simulink model "shell_elec_electric_vehicle"  (R2016b)
settings: Solver=FixedStepAuto  StartTime=0.0  StopTime=200  RelTol=1e-3  AbsTol=1e-3
PreLoadFcn:
  | % Simulation parameters
  | dt = 0.01;
  | 
  | % Battery cell parameters
  | ssc_lithium_cell_1RC_ini
  | 
  | % Motor parameters
  | max_torque = 220;
  | max_power = 50e3;
  | 
  | % Vehicle parameters
  | vehicle_mass = 1000;
  | wheel_radius = 0.25;
  | area = 5;
  | drag_coefficient = 0.25;
  | air_density = 1.225;
  | gravity = 9.81;
  | rolling_res_ratio = 0.015;
  | 
  | % Differential drive parameters
  | gear_ratio = 6;
  | 
  | % Simplified braking system parameters
  | force_max_pedal = 500;
  | braking_torque_to_pedal_force_ratio = -4;
  | 
  | % Vehicle controller parameters
  | hill_hold_max_speed = 0.5;
  | 
  | % Water properties for cooling circuit
  | load WaterProperties
values from neighbouring files (symbols this model uses):
  C1_LUT = [1913.6 12447 30609 ... (first row only)    [shell_elec_electric_vehicle_settings.m]
  Capacity_LUT = [28.0081 27.625 27.6392]    [shell_elec_electric_vehicle_settings.m]
  cell_mass = 1    [shell_elec_electric_vehicle_settings.m]
  Qe_init = 15.6845    [shell_elec_electric_vehicle_settings.m]
  R0_LUT = [0.0117 0.0085 0.009 ... (first row only)    [shell_elec_electric_vehicle_settings.m]
  R1_LUT = [0.0109 0.0029 0.0013 ... (first row only)    [shell_elec_electric_vehicle_settings.m]
  T_init = 293.15    [shell_elec_electric_vehicle_settings.m]
undefined symbols (not defined in the file or in its folder): DiscIntNeverNeededParam, sigbuilder_block
undefined symbols (not defined in the file): cell_Cp_heat, Em_LUT, SOC_LUT, Temperature_LUT
libraries: fl_lib x82, nesl_utility x12, LiBatteryElements_lib x4, elec_lib x2, instrumentlib x2, simulink_extras x1, simulink x1
Description:
  | Electric Vehicle Configured for HIL
  | 
  | This example shows an electric vehicle model suitable for
  | Hardware-In-the-Loop (HIL) deployment. Energy-based modeling
  | is used to avoid high-frequency switching, and solvers set for
  | fixed-step simulation.
  | 
  | The test run shows the vehicle accelerating to a steady speed up
  | an incline followed by a period of descent during which electrical
  | power is returned to the battery.
  | 
  | Copyright 2008-2016 The MathWorks, Inc.
settings Model: Creator=MathWorks  LastModifiedBy=eliya
settings SolverCC: InitialStep=1e-3
settings DataIOCC: LimitDataPoints=on  SaveFormat=Array  InspectSignalLogs=on
settings OptimizationCC: BlockReduction=off  BooleanDataType=off  LifeSpan=inf
settings DebuggingCC: SaveWithParameterizedLinksMsg=none  UnderspecifiedInitializationDetection=Classic  MergeDetectMultiDrivingBlocksExec=none  SignalResolutionControl=TryResolveAllWithWarning  AllowSymbolicDim=off  SFUnexpectedBacktrackingDiag=warning  SFNoUnconditionalDefaultTransitionDiag=warning  SFExecutionAtInitializationDiag=none
settings HardwareCC: ProdBitPerPointer=32  ProdBitPerSizeT=32  ProdBitPerPtrDiffT=32  ProdLargestAtomicFloat=None  ProdIntDivRoundTo=Undefined  ProdEndianess=Unspecified  ProdWordSize=32  ProdHWDeviceType=32-bit Generic  TargetUnknown=on
settings ModelReferenceCC: PropagateSignalLabelsOutOfModel=off
settings GRTTargetCC: TargetLangStandard=C89/C90 (ANSI)  GeneratePreprocessorConditionals=Disable all
settings ConfigComp: CovMetricSettings=dw  CovHtmlReporting=on  CovSaveCumulativeToWorkspaceVar=on  CovSaveSingleToWorkspaceVar=on  CovExternalEMLEnable=off  CovSFcnEnable=off
settings SimscapeCC: SimscapeLogType=all  SimscapeLogName=simlog_elec_electric_vehicle  SimscapeLogDataHistory=10000

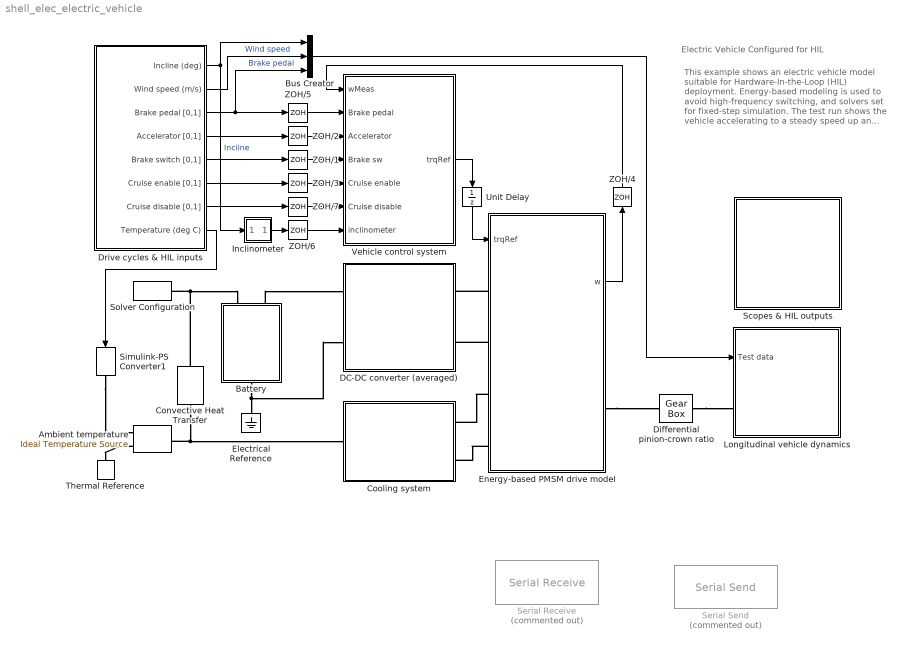
== system shell_elec_electric_vehicle ==
  note: Electric Vehicle Configured for HIL
  note: This example shows an electric vehicle model suitable for Hardware-In-the-Loop (HIL) deployment. Energy-based modeling is used to avoid high-frequency switching, and solvers set for fixed-step simulation.
      |
      | The test run shows the vehicle accelerating to a steady speed up an incline followed by a period of descent during which electrical power is returned to the battery.
  Ambient temperature : fl_lib/Thermal/Thermal Sources/Ideal Temperature Source
  Battery : Subsystem  mask(Lithium cell (one RC-branch equivalent circuit)){Nseries=50, Nparallel=10, Qe_init=Qe_init, T_init=T_init, Capacity_LUT=Capacity_LUT, Em_LUT=Em_LUT, R0_LUT=R0_LUT, R1_LUT=R1_LUT, C1_LUT=C1_LUT, cell_mass=cell_mass, cell_Cp_heat=cell_Cp_heat, SOC_LUT=SOC_LUT, Temperature_LUT=Temperature_LUT}
      mask prompts: Nseries "Number of series-connected cells"; Nparallel "Number of parallel sets of series-connected cells"; Qe_init "Initial cell charge deficit (A*hr)"; T_init "Initial cell temperature (K)"; Capacity_LUT "Capacity (A*hr, 1xN table)"; Em_LUT "Em open-circuit voltage, Em (volts, MxN table)"; R0_LUT "R0 terminal resistance (ohms, MxN table)"; R1_LUT "R1 cell resistance (ohms, MxN table)"; C1_LUT "C1 capacitance (farads, MxN table)"; cell_mass "Cell mass (kg)"; cell_Cp_heat "Cell specific heat (J/kg/K)"; SOC_LUT "SOC table breakpoints (Mx1 array)"; Temperature_LUT "Temperature table breakpoints (K, 1xN array)"
      mask Display:
      | % Battery icon
      | plot([2.5 1.3],[0 0])
      | plot([-0.6 -1.6 -1.6 -2.5],[0 0 -0.8 -0.8])
      | patch([1 1 -1 -1]*0.15+1.3,[-1 1 1 -1]*0.4,[0;0;0]);
      | patch([1 1 -1 -1]*0.15+0.0,[-1 1 1 -1]*0.4,[0;0;0]);
      | patch([1 1 -1 -1]*0.15+0.7,[-1 1 1 -1]*0.8,[0;0;0]);
      | patch([1 1 -1 -1]*0.15-0.6,[-1 1 1 -1]*0.8,[0;0;0]);
      | % Thermal port
      | plot([-1.6,-1.3],[1.2,1.2])
      | plot([-1.6,-1.3],[0.5,0.5])
      | plot([-1.6,-2.5],[0.8,0.8])
      | plot(0.2*sin(0:2*pi/50:2*pi)-1.6,0.35*cos(0:2*pi/50:2*pi)+0.85)
      | plot(0.2*sin(0:2*pi/50:pi)-1.3,0.35*cos(0:2*pi/50:pi)+0.85)
      | 
      | % Plot points to set plot range
      | color('white');plot(2.5,1.5);plot(-2.5,-1.5)
      | 
      | color('red')
      | port_label('LConn',1,'H')
      | port_label('LConn',2,'+')
      | port_label('RConn',1,'-')
  Bus Creator : BusCreator  Inputs=3
  Convective Heat Transfer : fl_lib/Thermal/Thermal Elements/Convective Heat Transfer  area=cell_area m^2  heat_tr_coeff=h_conv W/(m^2 * K)  Q_specify=off  Q_priority=High  Q=0 J/s  T_specify=off  T_priority=High  T=0 K
  Cooling system : Subsystem
  DC-DC converter (averaged) : Subsystem
  Differential pinion-crown ratio : fl_lib/Mechanical/Mechanisms/Gear Box  ratio=gear_ratio  t_in_specify=off  t_in_priority=High  t_in=0 N*m  t_out_specify=off  t_out_priority=High  t_out=0 N*m
  Drive cycles & HIL inputs : Subsystem  Tag=STV Subsys  LoadFcn=sigbuilder_block('load',[6 33 1428 678 ]);  StartFcn=sigbuilder_block('start');  StopFcn=sigbuilder_block('stop');  ClipboardFcn=sigbuilder_block('clipboard');  mask(Sigbuilder block){tuvar=[0:10]}
      mask help: Simulink:masks:SigbuilderBlock_MD
      mask init:
      | if ~strcmp(get_param(bdroot(gcbh),'SimulationStatus'),'stopped') tuvar = sigbuilder_block('maskInit'); end
      settings: CopyFcn=sigbuilder_block('copy');  DeleteFcn=sigbuilder_block('delete');  ModelCloseFcn=sigbuilder_block('modelClose');  PreSaveFcn=sigbuilder_block('preSave');  PauseFcn=sigbuilder_block('pause');  ContinueFcn=sigbuilder_block('continue');  NameChangeFcn=sigbuilder_block('namechange');  OpenFcn=sigbuilder_block('open',[6 33 1428 678 ]);  CloseFcn=sigbuilder_block('close');
      mask Display: plot(0, 0, 100, 100,[2, 2, 32, 32, 2], [68, 8, 8, 68, 68],[32, 2], [38, 38], [32, 19, 2],[53, 60, 44], [32, 17, 17, 2],[16, 16, 31, 31]);txt = getActiveGroup(gcbh);text(2, 100, txt,'verticalAlignment', 'top');
  Electrical Reference : fl_lib/Electrical/Electrical Elements/Electrical Reference
  Energy-based PMSM drive model : Subsystem  VariantControl=Variant1
  Inclinometer : Subsystem
  Longitudinal vehicle dynamics : Subsystem
  Scopes & HIL outputs : Subsystem
  Serial Receive : instrumentlib/Serial Receive  Commented=on  ComPortMenu=<Please select a port...>  ComPort=<Please select a port...>  Terminator=<none>  DataSize=[1 1]  DataType=uint8  EnableBlockingMode=on  ActionDataUnavailable=Output last received value  CustomValue=0  SampleTime=0.01
  Serial Send : instrumentlib/Serial Send  Commented=on  ComPortMenu=<Please select a port...>  ComPort=<Please select a port...>  Terminator=<none>  EnableBlockingMode=on
  Simulink-PS Converter1 : nesl_utility/Simulink-PS Converter  PhysicalDomain=network_engine_domain  SubClassName=ps_input  LeftPortType=input  RightPortType=output  PseudoPeriodic=off  Frequencies=[]  NoiseDistribution=none  NoiseParameters=[]  Unit=degC  AffineConversion=on  InputFiltering=off  SimscapeFilterOrder=1  InputFilterTimeConstant=.001  UdotUserProvided=1
  Solver Configuration : nesl_utility/Solver Configuration  PhysicalDomain=network_engine_domain  SubClassName=solver  LeftPortType=input  RightPortType=generic  Accelerate=off  Tones=[]  Harmonics=[]  SimulateNoise=off  Profile=off  UseLocalSampling=off  EnableSwitchedLinearOptims=on  FrequencyDomain=off  UseCCode=off  RelTol=0.001  AbsTol=1e-06  MinStep=1e-09  ToWorkspace=off  RevertToSquareIcSolve=off  NumHomotopyIterations=100  PhasorMode=off  PhasorModeNumHarmonics=1  OverrideAbsTol=off  DoDC=off  ResidualTolerance=1e-9  UseLocalSolver=on  LocalSolverChoice=NE_BACKWARD_EULER_ADVANCER  LocalSolverSampleTime=dt  DoFixedCost=on  MaxNonlinIter=3  MaxModeIter=2  LinearAlgebra=Sparse  DelaysMemoryBudget=1024  AutomaticFiltering=on  FilteringTimeConstant=0.001
  Thermal Reference : fl_lib/Thermal/Thermal Elements/Thermal Reference
  Unit Delay : UnitDelay  SampleTime=dt
  Vehicle control system : Subsystem
  ZOH/{1..7} (7 alike) : ZeroOrderHold  SampleTime=dt
  wires:
  Drive cycles & HIL inputs/8(Temperature (deg C)) -> Simulink-PS Converter1/1
  Drive cycles & HIL inputs/1(Incline (deg)) -> Bus Creator/1, Inclinometer/1(a)  "Incline"
  Drive cycles & HIL inputs/2(Wind speed (m/s)) -> Bus Creator/2  "Wind speed"
  ZOH/2/1 -> Vehicle control system/3(Accelerator)
  Drive cycles & HIL inputs/4(Accelerator [0,1]) -> ZOH/2/1
  ZOH/3/1 -> Vehicle control system/5(Cruise enable)
  Drive cycles & HIL inputs/6(Cruise enable [0,1]) -> ZOH/3/1
  ZOH/5/1 -> Vehicle control system/2(Brake pedal)
  ZOH/1/1 -> Vehicle control system/4(Brake sw)
  ZOH/6/1 -> Vehicle control system/7(inclinometer)
  ZOH/7/1 -> Vehicle control system/6(Cruise disable)
  Drive cycles & HIL inputs/3(Brake pedal [0,1]) -> ZOH/5/1, Bus Creator/3  "Brake pedal"
  ZOH/4/1 -> Vehicle control system/1(wMeas)
  Drive cycles & HIL inputs/5(Brake switch [0,1]) -> ZOH/1/1
  Drive cycles & HIL inputs/7(Cruise disable [0,1]) -> ZOH/7/1
  Inclinometer/1(y) -> ZOH/6/1
  Vehicle control system/1(trqRef) -> Unit Delay/1
  Unit Delay/1 -> Energy-based PMSM drive model/1(trqRef)
  Energy-based PMSM drive model/1(w) -> ZOH/4/1
  Bus Creator/1 -> Longitudinal vehicle dynamics/1(Test data)
  connections:
  Ambient temperature/RConn2 -- Thermal Reference/LConn1
  Simulink-PS Converter1/RConn1 -- Ambient temperature/RConn1
  Convective Heat Transfer/RConn1 -- Solver Configuration/RConn1 -- Battery/LConn1
  Battery/RConn1 -- DC-DC converter (averaged)/LConn2 -- Electrical Reference/LConn1
  Battery/LConn2 -- DC-DC converter (averaged)/LConn1
  Differential pinion-crown ratio/RConn1 -- Longitudinal vehicle dynamics/LConn1
  Energy-based PMSM drive model/LConn1 -- DC-DC converter (averaged)/RConn1
  Energy-based PMSM drive model/LConn2 -- DC-DC converter (averaged)/RConn2
  Energy-based PMSM drive model/RConn1 -- Differential pinion-crown ratio/LConn1
  Convective Heat Transfer/LConn1 -- Ambient temperature/LConn1 -- Cooling system/LConn1
  Energy-based PMSM drive model/LConn4 -- Cooling system/RConn2
  Energy-based PMSM drive model/LConn3 -- Cooling system/RConn1

== system shell_elec_electric_vehicle/Battery ==
  note: Scale up voltage drop to total of Ns series-connected cells
  Controlled Voltage Source : fl_lib/Electrical/Electrical Sources/Controlled Voltage Source
  Electrical model for Np parallel-connected cells : Subsystem
  Ns : fl_lib/Physical Signals/Functions/PS Gain  gain=Nseries
  Ns-1 : fl_lib/Physical Signals/Functions/PS Gain  gain=(Nseries-1)
  Thermal Model : Subsystem
  Voltage Sensor : fl_lib/Electrical/Electrical Sensors/Voltage Sensor
  - : PMIOPort  Tag=PMCPort  Port=1  Side=Right
  H : PMIOPort  Tag=PMCPort  Port=2  Side=Left
  + : PMIOPort  Tag=PMCPort  Port=3  Side=Left
  connections:
  Controlled Voltage Source/RConn2 -- -/RConn1
  Ns-1/RConn1 -- Controlled Voltage Source/RConn1
  +/RConn1 -- Electrical model for Np parallel-connected cells/RConn1 -- Voltage Sensor/LConn1
  Voltage Sensor/RConn1 -- Ns-1/LConn1
  Controlled Voltage Source/LConn1 -- Electrical model for Np parallel-connected cells/RConn2 -- Voltage Sensor/RConn2
  H/RConn1 -- Thermal Model/LConn2
  Thermal Model/RConn1 -- Electrical model for Np parallel-connected cells/LConn2
  Electrical model for Np parallel-connected cells/LConn1 -- Ns/LConn1
  Ns/RConn1 -- Thermal Model/LConn1

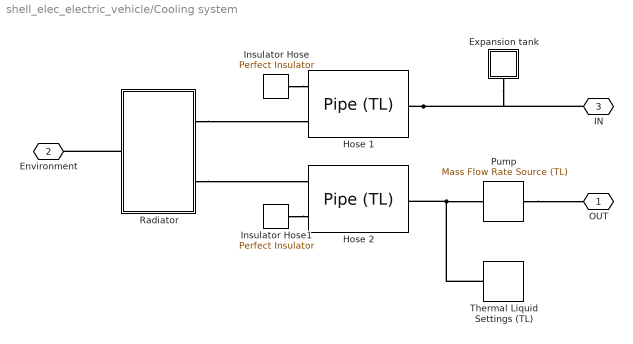
== system shell_elec_electric_vehicle/Cooling system ==
  Expansion tank : Subsystem
  Hose 1 : fl_lib/Thermal Liquid/Elements/Pipe (TL)  dynamic_compressibility=1  inertia=0  length=500 mm  area=pi*25^2 mm^2  Dh=50 mm  length_add=500 mm  roughness=1.5e-5 m  Re_lam=2e+3  Re_tur=4e+3  shape_factor=64  Nu_lam=3.66  p0=1 atm  T0=20 degC  mdot0=0.1 kg/s
  Hose 2 : fl_lib/Thermal Liquid/Elements/Pipe (TL)  dynamic_compressibility=1  inertia=0  length=500 mm  area=pi*25^2 mm^2  Dh=50 mm  length_add=500 mm  roughness=1.5e-5 m  Re_lam=2e+3  Re_tur=4e+3  shape_factor=64  Nu_lam=3.66  p0=1 atm  T0=20 degC  mdot0=0.1 kg/s
  Insulator Hose : fl_lib/Thermal/Thermal Elements/Perfect Insulator  T_specify=off  T_priority=High  T=0 K
  Insulator Hose1 : fl_lib/Thermal/Thermal Elements/Perfect Insulator  T_specify=off  T_priority=High  T=0 K
  Pump : fl_lib/Thermal Liquid/Sources/Mass Flow Rate Source (TL)  commanded_mass_flow=0.2 kg/s  area=pi*25^2 mm^2  length=1e-1 m
  Radiator : Subsystem
  Thermal Liquid Settings (TL) : fl_lib/Thermal Liquid/Utilities/Thermal Liquid Settings (TL)  pT_region_flag=0  T_min=273.16 K  T_max=373.16 K  p_min=0.1 bar  p_max=500 bar  T_TLU=T K  p_TLU=p Pa  pT_validity_TLU=ones(11, 12)  rho_TLU=rho kg/m^3  u_TLU=u J/g  nu_TLU=nu cm^2/s  cp_TLU=Cp J/K/g  k_TLU=k mW/m/K  beta_TLU=beta Pa  alpha_TLU=alpha 1/K  p_atm=1 atm
  OUT : PMIOPort  Port=1  Side=Right
  Environment : PMIOPort  Port=2  Side=Left
  IN : PMIOPort  Port=3  Side=Right
  connections:
  Insulator Hose1/LConn1 -- Hose 2/LConn2
  Insulator Hose/LConn1 -- Hose 1/LConn2
  Radiator/LConn1 -- Environment/RConn1
  Thermal Liquid Settings (TL)/RConn1 -- Pump/LConn1 -- Hose 2/RConn1
  Radiator/RConn1 -- Hose 1/LConn1
  Radiator/RConn2 -- Hose 2/LConn1
  Pump/RConn1 -- OUT/RConn1
  Hose 1/RConn1 -- Expansion tank/RConn1 -- IN/RConn1

== system shell_elec_electric_vehicle/DC-DC converter (averaged) ==
  Battery sensors : Subsystem
  DC-DC Converter : elec_lib/Sources/DC-DC Converter  v_ref=400 V  P_rated=60 kW  droop_param=2  droop=0.1 V/A  droop_percent=1  reversible=1  efficiency=98  P_fixed=100 W  model_dynamics=0  tau=0.02 s  v_ini=400 V  i1_max=1000 A  fault_condition=1  fault_threshold=0.5  R_fixed=100 Ohm  R_out=0.1 Ohm  fault_sign=1
  No faults : fl_lib/Physical Signals/Sources/PS Constant  constant=0
  Resistor : fl_lib/Electrical/Electrical Elements/Resistor  R=0.002 Ohm  i_specify=off  i_priority=None  i=0 A  v_specify=off  v_priority=None  v=0 V
  Vbat+ : PMIOPort  Port=1  Side=Left
  V+ : PMIOPort  Tag=PMCPort  Port=2  Side=Right
  Vbat- : PMIOPort  Port=3  Side=Left
  V- : PMIOPort  Tag=PMCPort  Port=4  Side=Right
  connections:
  No faults/RConn1 -- DC-DC Converter/LConn3
  DC-DC Converter/RConn2 -- V-/RConn1 -- DC-DC Converter/LConn2 -- Battery sensors/LConn1 -- Vbat-/RConn1
  Vbat+/RConn1 -- Battery sensors/RConn1
  Battery sensors/RConn2 -- DC-DC Converter/LConn1
  DC-DC Converter/RConn1 -- Resistor/LConn1
  Resistor/RConn1 -- V+/RConn1

== system shell_elec_electric_vehicle/Drive cycles & HIL inputs ==
  Demux : Demux  Tag=STV Demux  Outputs=8
  FromWs : FromWorkspace  Tag=STV FromWs  VariableName=tuvar  SampleTime=0.01
      SigBuilderData=|
      | common.afterFinalStr = 'Extrapolate'
      | common.sampleTime = '0.01'
      | dataSet.timeRange = [0 200]
      | dataSet.name = 'Test 1'
      | sbobj.Name = 'Signal Builder'
      | sbobj.Groups.Name = 'Test 1'
      | sbobj.Groups.Signals(1).Name = 'Incline (deg)'
      | sbobj.Groups.Signals(1).XData = [0 100 200]
      | sbobj.Groups.Signals(1).YData = [0 0 0]
      | sbobj.Groups.Signals(2).Name = 'Wind speed (m/s)'
      | sbobj.Groups.Signals(2).XData = [0 200]
      | sbobj.Groups.Signals(2).YData = [0 0]
      | sbobj.Groups.Signals(3).Name = 'Brake pedal [0,1]'
      | sbobj.Groups.Signals(3).XData = [0 180 180 200]
      | sbobj.Groups.Signals(3).YData = [0 0 1 1]
      | sbobj.Groups.Signals(4).Name = 'Accelerator [0,1]'
      | sbobj.Groups.Signals(4).XData = [0 0.1 0.3 7.5 50 200]
      | sbobj.Groups.Signals(4).YData = [0 0 0 1 0 0]
      | sbobj.Groups.Signals(5).Name = 'Brake switch [0,1]'
      | sbobj.Groups.Signals(5).XData = [0 180 180 200]
      | sbobj.Groups.Signals(5).YData = [0 0 1 1]
      | sbobj.Groups.Signals(6).Name = 'Cruise enable [0,1]'
      | sbobj.Groups.Signals(6).XData = [0 8 8 10 10 200]
      | sbobj.Groups.Signals(6).YData = [0 0 1 1 0 0]
      | sbobj.Groups.Signals(7).Name = 'Cruise disable [0,1]'
      | sbobj.Groups.Signals(7).XData = [0 200]
      | sbobj.Groups.Signals(7).YData = [0 0]
      | sbobj.Groups.Signals(8).Name = 'Temperature (deg C)'
      | sbobj.Groups.Signals(8).XData = [0 200]
      | sbobj.Groups.Signals(8).YData = [25 25]
      | sbobj.Groups.TimeRange = [0 200]
  Incline (deg) : Outport  Tag=STV Outport
  Wind speed (m/s) : Outport  Tag=STV Outport  Port=2
  Brake pedal [0,1] : Outport  Tag=STV Outport  Port=3
  Accelerator [0,1] : Outport  Tag=STV Outport  Port=4
  Brake switch [0,1] : Outport  Tag=STV Outport  Port=5
  Cruise enable [0,1] : Outport  Tag=STV Outport  Port=6
  Cruise disable [0,1] : Outport  Tag=STV Outport  Port=7
  Temperature (deg C) : Outport  Tag=STV Outport  Port=8
  wires:
  FromWs/1 -> Demux/1
  Demux/1 -> Incline (deg)/1
  Demux/2 -> Wind speed (m/s)/1
  Demux/3 -> Brake pedal [0,1]/1
  Demux/4 -> Accelerator [0,1]/1
  Demux/5 -> Brake switch [0,1]/1
  Demux/6 -> Cruise enable [0,1]/1
  Demux/7 -> Cruise disable [0,1]/1
  Demux/8 -> Temperature (deg C)/1

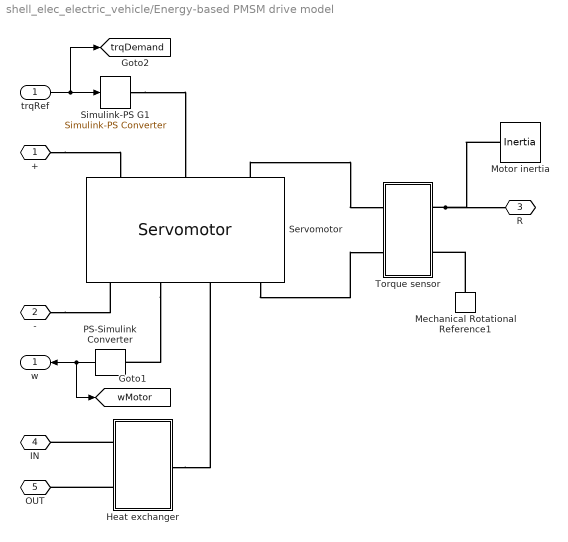
== system shell_elec_electric_vehicle/Energy-based PMSM drive model ==
  trqRef : Inport
  Heat exchanger : Subsystem
  Mechanical Rotational Reference1 : fl_lib/Mechanical/Rotational Elements/Mechanical Rotational Reference
  Motor inertia : fl_lib/Mechanical/Rotational Elements/Inertia  inertia=0.02 kg*m^2  w_specify=on  w_priority=High  w=0 rpm  t_specify=off  t_priority=High  t=0 N*m
  PS-Simulink Converter : nesl_utility/PS-Simulink Converter  PhysicalDomain=network_engine_domain  SubClassName=ps_output  LeftPortType=input  RightPortType=output  PseudoPeriodic=off  Frequencies=[]  Unit=rad/s  AffineConversion=off
  Servomotor : elec_lib/Actuators & Drivers/Rotational Actuators/Servomotor  torque_speed_param=2  w_t=[ 0 3.75e+3 7.5e+3 8e+3 ] rpm  T_t=[max_torque max_torque max_torque 0] N*m  torque_max=max_torque N*m  power_max=max_power W  Tc=0.02 s  losses_param=1  eff=96  w_eff=1500 rpm  T_eff=50 N*m  Piron=200 W  Pbase=0 W  w_eff_vec=[-8000 -4000 0 4000 8000] rpm  T_eff_vec=[0 0.03 0.06 0.09] N*m  losses_mat=[1.49 1.67 2.21 3.10; 0.42 0.69 1.14 2.03; 0.06 0.24 0.78 1.68; 0.42 0.69 1.14 2.03; 1.49 1.67 2.21 3.10] W  efficiency_mat=[95 95 95 95; 95 95 95 95; 95 95 95 95; 95 95 95 95; 95 95 95 95]  Res=0 Ohm  J=0 kg*m^2  lam=1e-5 N*m/(rad/s)  speed0=0 rpm  alpha=0.00393 1/K  Tmeas=25 degC  Tmeas2=125 degC  losses_mat_T2=[1.49 1.74 2.49 3.74;0.42 0.67 1.42 2.67;0.06 0.31 1.06 2.31;0.42 0.67 1.42 2.67;1.49 1.74 2.49 3.74] W  efficiency_mat_T2=[95 95 95 95; 95 95 95 95; 95 95 95 95; 95 95 95 95; 95 95 95 95]  thermal_mass=1500 J/K  initial_temperature=20 degC  fault_condition=1  fault_threshold=0.5
  Simulink-PS G1 : nesl_utility/Simulink-PS Converter  PhysicalDomain=network_engine_domain  SubClassName=ps_input  LeftPortType=input  RightPortType=output  PseudoPeriodic=off  Frequencies=[]  NoiseDistribution=none  NoiseParameters=[]  Unit=1  AffineConversion=off  InputFiltering=off  SimscapeFilterOrder=1  InputFilterTimeConstant=1e-6  UdotUserProvided=1
  Torque sensor : Subsystem
  + : PMIOPort  Port=1  Side=Left
  - : PMIOPort  Port=2  Side=Left
  R : PMIOPort  Port=3  Side=Right
  IN : PMIOPort  Port=4  Side=Left
  OUT : PMIOPort  Port=5  Side=Left
  w : Outport
  tag scope: trqDemand=global, wMotor=global
  wires:
  PS-Simulink Converter/1 -> w/1, [wMotor]
  trqRef/1 -> Simulink-PS G1/1, [trqDemand]
  connections:
  Servomotor/RConn2 -- PS-Simulink Converter/LConn1
  Simulink-PS G1/RConn1 -- Servomotor/LConn2
  -/RConn1 -- Servomotor/RConn1
  +/RConn1 -- Servomotor/LConn1
  Heat exchanger/LConn1 -- IN/RConn1
  Heat exchanger/LConn2 -- OUT/RConn1
  Heat exchanger/RConn1 -- Servomotor/RConn3
  Servomotor/LConn3 -- Torque sensor/LConn1
  Servomotor/RConn4 -- Torque sensor/LConn2
  Mechanical Rotational Reference1/LConn1 -- Torque sensor/RConn2
  Torque sensor/RConn1 -- R/RConn1 -- Motor inertia/LConn1

== system shell_elec_electric_vehicle/Inclinometer ==
  a : Inport
  Trigonometric Function : Trigonometry
  d2r : Gain  Gain=pi/180
  g : Gain  Gain=gravity
  y : Outport
  wires:
  Trigonometric Function/1 -> g/1
  a/1 -> d2r/1
  d2r/1 -> Trigonometric Function/1
  g/1 -> y/1

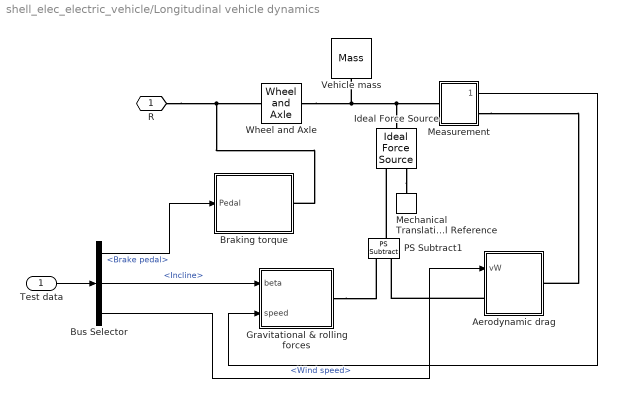
== system shell_elec_electric_vehicle/Longitudinal vehicle dynamics ==
  Test data : Inport
  Aerodynamic drag : Subsystem
  Braking torque : Subsystem
  Bus Selector : BusSelector  OutputSignals=Brake pedal,Incline,Wind speed
  Gravitational & rolling forces : Subsystem
  Ideal Force Source : fl_lib/Mechanical/Mechanical Sources/Ideal Force Source
  Measurement : Subsystem
  Mechanical Translational Reference : fl_lib/Mechanical/Translational Elements/Mechanical Translational Reference
  PS Subtract1 : fl_lib/Physical Signals/Functions/PS Subtract
  Vehicle mass : fl_lib/Mechanical/Translational Elements/Mass  mass=vehicle_mass kg  v_specify=off  v_priority=High  v=0 m/s  f_specify=off  f_priority=High  f=0 N
  Wheel and Axle : fl_lib/Mechanical/Mechanisms/Wheel and Axle  R=wheel_radius m  or=1  t_specify=off  t_priority=High  t=0 N*m  f_specify=off  f_priority=High  f=0 N
  R : PMIOPort  Port=1  Side=Left
  wires:
  Test data/1 -> Bus Selector/1
  Bus Selector/1 -> Braking torque/1(Pedal)  "<Brake pedal>"
  Bus Selector/2 -> Gravitational & rolling forces/1(beta)  "<Incline>"
  Bus Selector/3 -> Aerodynamic drag/1(vW)  "<Wind speed>"
  Measurement/1(speed) -> Gravitational & rolling forces/2(speed)
  connections:
  Ideal Force Source/RConn2 -- Mechanical Translational Reference/LConn1
  R/RConn1 -- Braking torque/RConn1 -- Wheel and Axle/LConn1
  PS Subtract1/RConn1 -- Ideal Force Source/RConn1
  Gravitational & rolling forces/RConn1 -- PS Subtract1/LConn1
  Aerodynamic drag/LConn1 -- PS Subtract1/LConn2
  Wheel and Axle/RConn1 -- Measurement/LConn1 -- Ideal Force Source/LConn1 -- Vehicle mass/LConn1
  Measurement/RConn1 -- Aerodynamic drag/RConn1

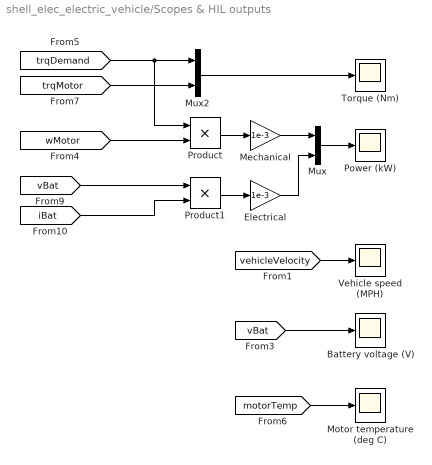
== system shell_elec_electric_vehicle/Scopes & HIL outputs ==
  " Electrical " : Gain  Gain=1e-3
  Battery voltage (V) : Scope
  Mechanical : Gain  Gain=1e-3
  Motor temperature (deg C) : Scope
  Mux : Mux  Inputs=2
  Mux2 : Mux  Inputs=2
  Power (kW) : Scope
  Product : Product
  Product1 : Product
  Torque (Nm) : Scope
  Vehicle speed (MPH) : Scope
  wires:
  [wMotor] -> Product/2
  [trqDemand] -> Product/1, Mux2/1
  [vehicleVelocity] -> Vehicle speed (MPH)/1
  [vBat] -> Battery voltage (V)/1
  Product/1 -> Mechanical/1
  [motorTemp] -> Motor temperature (deg C)/1
  [trqMotor] -> Mux2/2
  [vBat] -> Product1/1
  [iBat] -> Product1/2
  Product1/1 -> " Electrical "/1
  Mechanical/1 -> Mux/1
  " Electrical "/1 -> Mux/2
  Mux/1 -> Power (kW)/1
  Mux2/1 -> Torque (Nm)/1

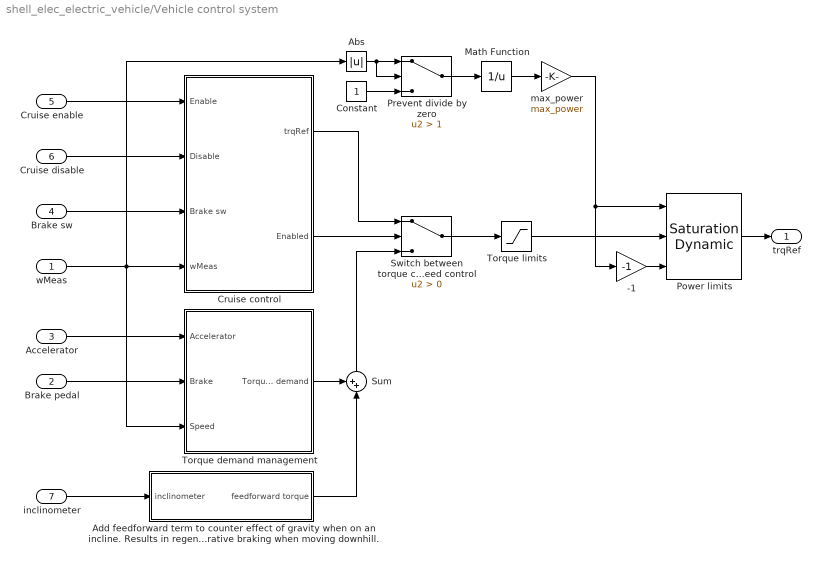
== system shell_elec_electric_vehicle/Vehicle control system ==
  wMeas : Inport
  Brake pedal : Inport  Port=2
  Accelerator : Inport  Port=3
  Brake sw : Inport  Port=4
  Cruise enable : Inport  Port=5
  Cruise disable : Inport  Port=6
  inclinometer : Inport  Port=7
  -1 : Gain  Gain=-1
  Abs : Abs
  Add feedforward term to counter effect of gravity when on an incline. Results in regenerative braking when moving downhill. : Subsystem
  Constant : Constant
  Cruise control : Subsystem
  Math Function : Math  Operator=reciprocal  SaturateOnIntegerOverflow=on
  Power limits : simulink/Discontinuities/Saturation Dynamic  OutMin=[]  OutMax=[]  OutDataTypeStr=Inherit: Same as second input  OutDataType=fixdt(1, 16)  OutScaling=2^-10  DoSatur=off
  Prevent divide by zero : Switch  Criteria=u2 > Threshold  Threshold=1
  Sum : Sum  Inputs=++|
  Switch between torque control and speed control : Switch  Criteria=u2 > Threshold
  Torque limits : Saturate  UpperLimit=max_torque  LowerLimit=-max_torque
  Torque demand management : Subsystem
  max_power : Gain  Gain=max_power
  trqRef : Outport
  wires:
  Switch between torque control and speed control/1 -> Torque limits/1
  Cruise enable/1 -> Cruise control/1(Enable)
  wMeas/1 -> Abs/1, Torque demand management/3(Speed), Cruise control/4(wMeas)
  Cruise control/1(trqRef) -> Switch between torque control and speed control/1
  Cruise control/2(Enabled) -> Switch between torque control and speed control/2
  Cruise disable/1 -> Cruise control/2(Disable)
  Brake sw/1 -> Cruise control/3(Brake sw)
  Accelerator/1 -> Torque demand management/1(Accelerator)
  Brake pedal/1 -> Torque demand management/2(Brake)
  inclinometer/1 -> Add feedforward term to counter effect of gravity when on an incline. Results in regenerative braking when moving downhill./1(inclinometer)
  Torque demand management/1(Torque demand) -> Sum/1
  Sum/1 -> Switch between torque control and speed control/3
  Add feedforward term to counter effect of gravity when on an incline. Results in regenerative braking when moving downhill./1(feedforward torque) -> Sum/2
  Torque limits/1 -> Power limits/2
  Power limits/1 -> trqRef/1
  Math Function/1 -> max_power/1
  max_power/1 -> Power limits/1, -1/1
  Prevent divide by zero/1 -> Math Function/1
  Constant/1 -> Prevent divide by zero/3
  Abs/1 -> Prevent divide by zero/2, Prevent divide by zero/1
  -1/1 -> Power limits/3

== system shell_elec_electric_vehicle/Battery/Electrical model for Np parallel-connected cells ==
  C1 : LiBatteryElements_lib/C_table  C_Table=C1_LUT*Nparallel F  SOC_Table=SOC_LUT  Temp_Table=Temperature_LUT K  v0=0 V
  Em_table : LiBatteryElements_lib/Em_table  C_Table=Capacity_LUT*Nparallel hr*A  Em_Table=Em_LUT V  SOC_Table=SOC_LUT  Temp_Table=Temperature_LUT K  Qinit=Qe_init*Nparallel hr*A
  Power Sum : fl_lib/Physical Signals/Functions/PS Add
  R0 : LiBatteryElements_lib/R_table  R_Table=R0_LUT/Nparallel Ohm  SOC_Table=SOC_LUT  Temp_Table=Temperature_LUT K
  R1 : LiBatteryElements_lib/R_table  R_Table=R1_LUT/Nparallel Ohm  SOC_Table=SOC_LUT  Temp_Table=Temperature_LUT K
  + : PMIOPort  Port=1  Side=Right
  - : PMIOPort  Port=2  Side=Right
  Ploss : PMIOPort  Port=3  Side=Left
  T : PMIOPort  Port=4  Side=Left
  connections:
  Ploss/RConn1 -- Power Sum/RConn1
  +/RConn1 -- R0/RConn1
  R0/LConn2 -- Em_table/RConn2 -- T/RConn1 -- R1/LConn2 -- C1/LConn2
  Em_table/LConn1 -- C1/LConn1 -- R1/LConn1
  R1/RConn2 -- Power Sum/LConn2
  R0/RConn2 -- Power Sum/LConn1
  R1/RConn1 -- C1/RConn1 -- R0/LConn1
  Em_table/RConn1 -- -/RConn1
  R0/LConn3 -- Em_table/LConn3 -- R1/LConn3 -- C1/LConn3

== system shell_elec_electric_vehicle/Battery/Thermal Model ==
  Battery thermal mass : fl_lib/Thermal/Thermal Elements/Thermal Mass  mass=cell_mass*Nseries*Nparallel kg  sp_heat=cell_Cp_heat J/kg/K  T_specify=on  T_priority=High  T=T_init K  Q_specify=off  Q_priority=High  Q=0 J/s
  Ideal Temperature Sensor : fl_lib/Thermal/Thermal Sensors/Ideal Temperature Sensor
  Ideal Heat Flow Source : fl_lib/Thermal/Thermal Sources/Ideal Heat Flow Source
  Thermal Reference1 : fl_lib/Thermal/Thermal Elements/Thermal Reference
  Thermal Reference2 : fl_lib/Thermal/Thermal Elements/Thermal Reference
  PlossTotal : PMIOPort  Tag=PMCPort  Port=1  Side=Left
  H : PMIOPort  Tag=PMCPort  Port=2  Side=Left
  T : PMIOPort  Tag=PMCPort  Port=3  Side=Right
  connections:
  Thermal Reference2/LConn1 -- Ideal Temperature Sensor/RConn1
  Ideal Temperature Sensor/RConn2 -- T/RConn1
  Thermal Reference1/LConn1 -- Ideal Heat Flow Source/RConn2
  Ideal Temperature Sensor/LConn1 -- H/RConn1 -- Battery thermal mass/LConn1 -- Ideal Heat Flow Source/LConn1
  Ideal Heat Flow Source/RConn1 -- PlossTotal/RConn1

== system shell_elec_electric_vehicle/Cooling system/Expansion tank ==
  Air stiffness : fl_lib/Mechanical/Translational Elements/Translational Spring  spr_rate=1e3 N/m  v_specify=off  v_priority=High  v=0 m/s  f_specify=on  f_priority=Low  f=0 N  x_specify=off  x_priority=High  x=0 m
  Local Restriction (TL) : fl_lib/Thermal Liquid/Elements/Local Restriction (TL)  restriction_area=pi*10^2 mm^2  area=pi*11^2 mm^2  length=1e-1 m  Cd=0.7  pressure_recovery=0  Re_c=12
  Mechanical Translational Reference : fl_lib/Mechanical/Translational Elements/Mechanical Translational Reference
  Mechanical Translational Reference1 : fl_lib/Mechanical/Translational Elements/Mechanical Translational Reference
  Perfect Insulator : fl_lib/Thermal/Thermal Elements/Perfect Insulator  T_specify=off  T_priority=High  T=0 K
  Translational Mechanical Converter (TL) : fl_lib/Thermal Liquid/Elements/Translational Mechanical Converter (TL)  mech_orientation=1  interface_area=pi*50^2 mm^2  x0=200 mm  dead_volume=0.001 m^3  environment_spec=1  environment_pressure=0.101325 MPa  dynamic_compressibility=0  T0=20 degC  p0=1 atm
  A : PMIOPort  Port=1  Side=Right
  connections:
  Air stiffness/RConn1 -- Mechanical Translational Reference1/LConn1
  Local Restriction (TL)/RConn1 -- Translational Mechanical Converter (TL)/LConn1
  Mechanical Translational Reference/LConn1 -- Translational Mechanical Converter (TL)/LConn2
  Perfect Insulator/LConn1 -- Translational Mechanical Converter (TL)/LConn3
  Air stiffness/LConn1 -- Translational Mechanical Converter (TL)/RConn1
  A/RConn1 -- Local Restriction (TL)/LConn1

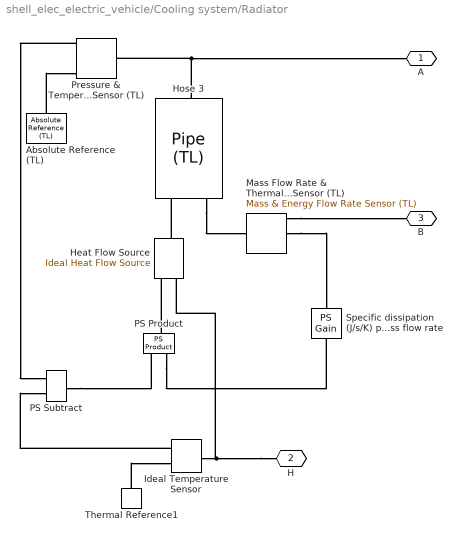
== system shell_elec_electric_vehicle/Cooling system/Radiator ==
  Absolute Reference (TL) : fl_lib/Thermal Liquid/Elements/Absolute Reference (TL)
  Heat Flow Source : fl_lib/Thermal/Thermal Sources/Ideal Heat Flow Source
  Hose 3 : fl_lib/Thermal Liquid/Elements/Pipe (TL)  dynamic_compressibility=1  inertia=0  length=2000 mm  area=pi*25^2 mm^2  Dh=50 mm  length_add=500 mm  roughness=1.5e-5 m  Re_lam=2e+3  Re_tur=4e+3  shape_factor=64  Nu_lam=3.66  p0=1 atm  T0=20 degC  mdot0=0.1 kg/s
  Ideal Temperature Sensor : fl_lib/Thermal/Thermal Sensors/Ideal Temperature Sensor
  Mass Flow Rate & Thermal Flux Sensor (TL) : fl_lib/Thermal Liquid/Sensors/Mass & Energy Flow Rate Sensor (TL)
  PS Product : fl_lib/Physical Signals/Functions/PS Product
  PS Subtract : fl_lib/Physical Signals/Functions/PS Subtract
  Pressure & Temperature Sensor (TL) : fl_lib/Thermal Liquid/Sensors/Pressure & Temperature Sensor (TL)
  Specific dissipation (J/s/K) per unit mass flow rate : fl_lib/Physical Signals/Functions/PS Gain  gain=100
  Thermal Reference1 : fl_lib/Thermal/Thermal Elements/Thermal Reference
  A : PMIOPort  Port=1  Side=Right
  H : PMIOPort  Port=2  Side=Left
  B : PMIOPort  Port=3  Side=Right
  connections:
  Heat Flow Source/LConn1 -- Hose 3/LConn2
  Mass Flow Rate & Thermal Flux Sensor (TL)/RConn2 -- Specific dissipation (J/s/K) per unit mass flow rate/LConn1
  PS Subtract/RConn1 -- PS Product/LConn1
  H/RConn1 -- Heat Flow Source/RConn2 -- Ideal Temperature Sensor/LConn1
  Hose 3/RConn1 -- A/RConn1 -- Pressure & Temperature Sensor (TL)/LConn1
  Hose 3/LConn1 -- Mass Flow Rate & Thermal Flux Sensor (TL)/LConn1
  Mass Flow Rate & Thermal Flux Sensor (TL)/RConn1 -- B/RConn1
  Thermal Reference1/LConn1 -- Ideal Temperature Sensor/RConn1
  Absolute Reference (TL)/LConn1 -- Pressure & Temperature Sensor (TL)/RConn1
  PS Product/RConn1 -- Heat Flow Source/RConn1
  Ideal Temperature Sensor/RConn2 -- PS Subtract/LConn1
  Pressure & Temperature Sensor (TL)/RConn3 -- PS Subtract/LConn2
  PS Product/LConn2 -- Specific dissipation (J/s/K) per unit mass flow rate/RConn1

== system shell_elec_electric_vehicle/DC-DC converter (averaged)/Battery sensors ==
  Current Sensor : fl_lib/Electrical/Electrical Sensors/Current Sensor
  PS-Simulink Converter : nesl_utility/PS-Simulink Converter  PhysicalDomain=network_engine_domain  SubClassName=ps_output  LeftPortType=input  RightPortType=output  PseudoPeriodic=off  Frequencies=[]  Unit=V  AffineConversion=off
  PS-Simulink Converter1 : nesl_utility/PS-Simulink Converter  PhysicalDomain=network_engine_domain  SubClassName=ps_output  LeftPortType=input  RightPortType=output  PseudoPeriodic=off  Frequencies=[]  Unit=A  AffineConversion=off
  Voltage Sensor : fl_lib/Electrical/Electrical Sensors/Voltage Sensor
  +1 : PMIOPort  Port=1  Side=Right
  - : PMIOPort  Port=2  Side=Left
  +2 : PMIOPort  Port=3  Side=Right
  tag scope: iBat=global, vBat=global
  wires:
  PS-Simulink Converter/1 -> [vBat]
  PS-Simulink Converter1/1 -> [iBat]
  connections:
  Voltage Sensor/RConn2 -- -/RConn1
  Voltage Sensor/LConn1 -- Current Sensor/LConn1 -- +1/RConn1
  Voltage Sensor/RConn1 -- PS-Simulink Converter/LConn1
  Current Sensor/RConn2 -- +2/RConn1
  Current Sensor/RConn1 -- PS-Simulink Converter1/LConn1

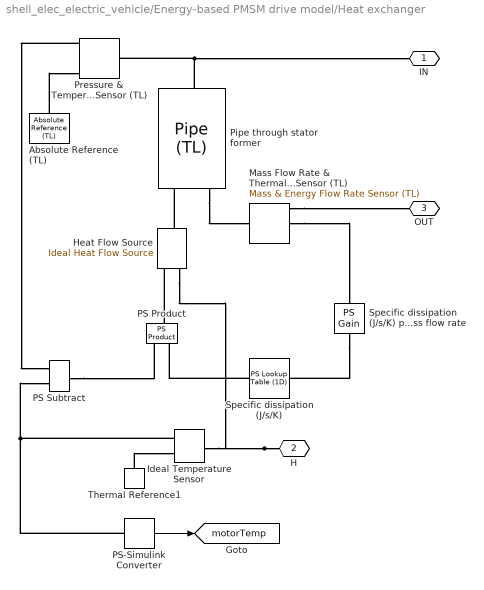
== system shell_elec_electric_vehicle/Energy-based PMSM drive model/Heat exchanger ==
  Absolute Reference (TL) : fl_lib/Thermal Liquid/Elements/Absolute Reference (TL)
  Heat Flow Source : fl_lib/Thermal/Thermal Sources/Ideal Heat Flow Source
  Ideal Temperature Sensor : fl_lib/Thermal/Thermal Sensors/Ideal Temperature Sensor
  Mass Flow Rate & Thermal Flux Sensor (TL) : fl_lib/Thermal Liquid/Sensors/Mass & Energy Flow Rate Sensor (TL)
  PS Product : fl_lib/Physical Signals/Functions/PS Product
  PS Subtract : fl_lib/Physical Signals/Functions/PS Subtract
  PS-Simulink Converter : nesl_utility/PS-Simulink Converter  PhysicalDomain=network_engine_domain  SubClassName=ps_output  LeftPortType=input  RightPortType=output  PseudoPeriodic=off  Frequencies=[]  Unit=degC  AffineConversion=on
  Pipe through stator former : fl_lib/Thermal Liquid/Elements/Pipe (TL)  dynamic_compressibility=1  inertia=0  length=400 mm  area=pi*25^2 mm^2  Dh=50 mm  length_add=500 mm  roughness=1.5e-5 m  Re_lam=2e+3  Re_tur=4e+3  shape_factor=64  Nu_lam=3.66  p0=1 atm  T0=20 degC  mdot0=0.1 kg/s
  Pressure & Temperature Sensor (TL) : fl_lib/Thermal Liquid/Sensors/Pressure & Temperature Sensor (TL)
  Specific dissipation (J/s/K) : fl_lib/Physical Signals/Lookup Tables/PS Lookup Table (1D)  x="[0 0.2 0.4  0.7  1 1.2  1.4  2.5 ]"  f=100 * [0 0.5 0.75 0.92 1 1.02 1.03 1.04]  interp_method=1  extrap_method=1
  Specific dissipation (J/s/K) per unit mass flow rate : fl_lib/Physical Signals/Functions/PS Gain  gain=100
  Thermal Reference1 : fl_lib/Thermal/Thermal Elements/Thermal Reference
  IN : PMIOPort  Port=1  Side=Left
  H : PMIOPort  Port=2  Side=Right
  OUT : PMIOPort  Port=3  Side=Left
  tag scope: motorTemp=global
  wires:
  PS-Simulink Converter/1 -> [motorTemp]
  connections:
  Heat Flow Source/LConn1 -- Pipe through stator former/LConn2
  PS Subtract/RConn1 -- PS Product/LConn1
  Pipe through stator former/RConn1 -- Pressure & Temperature Sensor (TL)/LConn1 -- IN/RConn1
  Pipe through stator former/LConn1 -- Mass Flow Rate & Thermal Flux Sensor (TL)/LConn1
  Specific dissipation (J/s/K)/RConn1 -- PS Product/LConn2
  H/RConn1 -- Heat Flow Source/RConn2 -- Ideal Temperature Sensor/LConn1
  Mass Flow Rate & Thermal Flux Sensor (TL)/RConn1 -- OUT/RConn1
  Thermal Reference1/LConn1 -- Ideal Temperature Sensor/RConn1
  Absolute Reference (TL)/LConn1 -- Pressure & Temperature Sensor (TL)/RConn1
  PS Product/RConn1 -- Heat Flow Source/RConn1
  Ideal Temperature Sensor/RConn2 -- PS-Simulink Converter/LConn1 -- PS Subtract/LConn1
  Pressure & Temperature Sensor (TL)/RConn3 -- PS Subtract/LConn2
  Mass Flow Rate & Thermal Flux Sensor (TL)/RConn2 -- Specific dissipation (J/s/K) per unit mass flow rate/LConn1
  Specific dissipation (J/s/K) per unit mass flow rate/RConn1 -- Specific dissipation (J/s/K)/LConn1

== system shell_elec_electric_vehicle/Energy-based PMSM drive model/Torque sensor ==
  Ideal Torque Sensor : fl_lib/Mechanical/Mechanical Sensors/Ideal Torque Sensor
  PS-Simulink Converter2 : nesl_utility/PS-Simulink Converter  PhysicalDomain=network_engine_domain  SubClassName=ps_output  LeftPortType=input  RightPortType=output  PseudoPeriodic=off  Frequencies=[]  Unit=N*m  AffineConversion=off
  1L : PMIOPort  Port=1  Side=Left
  2L : PMIOPort  Port=2  Side=Left
  1R : PMIOPort  Port=3  Side=Right
  2R : PMIOPort  Port=4  Side=Right
  tag scope: trqMotor=global
  wires:
  PS-Simulink Converter2/1 -> [trqMotor]
  connections:
  1R/RConn1 -- Ideal Torque Sensor/RConn1
  2R/RConn1 -- 2L/RConn1
  1L/RConn1 -- Ideal Torque Sensor/LConn1
  Ideal Torque Sensor/RConn2 -- PS-Simulink Converter2/LConn1

== system shell_elec_electric_vehicle/Longitudinal vehicle dynamics/Aerodynamic drag ==
  vW : Inport
  0.5*Cd*density*area : fl_lib/Physical Signals/Functions/PS Gain  gain=0.5*drag_coefficient*air_density*area
  PS Product : fl_lib/Physical Signals/Functions/PS Product
  PS Subtract : fl_lib/Physical Signals/Functions/PS Subtract
  Simulink-PS Converter2 : nesl_utility/Simulink-PS Converter  PhysicalDomain=network_engine_domain  SubClassName=ps_input  LeftPortType=input  RightPortType=output  PseudoPeriodic=off  Frequencies=[]  NoiseDistribution=none  NoiseParameters=[]  Unit=N*m  AffineConversion=off  InputFiltering=off  SimscapeFilterOrder=1  InputFilterTimeConstant=0.001  UdotUserProvided=1
  u^2 : fl_lib/Physical Signals/Functions/PS Math Function  fcn_choice=7
  y=tanh(x) : Subsystem
  vV : PMIOPort  Port=1  Side=Right
  F : PMIOPort  Port=2  Side=Left
  wires:
  vW/1 -> Simulink-PS Converter2/1
  connections:
  vV/RConn1 -- PS Subtract/LConn1
  Simulink-PS Converter2/RConn1 -- PS Subtract/LConn2
  u^2/LConn1 -- y=tanh(x)/LConn1 -- PS Subtract/RConn1
  0.5*Cd*density*area/LConn1 -- u^2/RConn1
  0.5*Cd*density*area/RConn1 -- PS Product/LConn2
  PS Product/RConn1 -- F/RConn1
  y=tanh(x)/RConn1 -- PS Product/LConn1

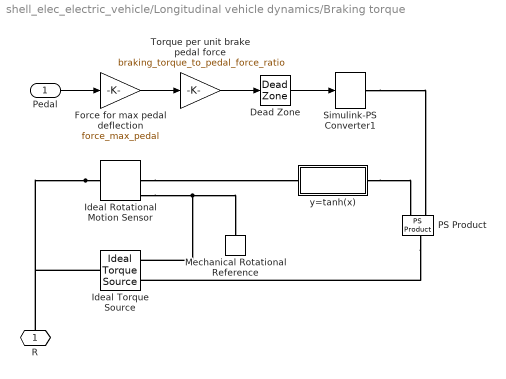
== system shell_elec_electric_vehicle/Longitudinal vehicle dynamics/Braking torque ==
  Pedal : Inport
  Dead Zone : DeadZone  LowerValue=-max_torque*gear_ratio  UpperValue=max_torque*gear_ratio  SaturateOnIntegerOverflow=on
  Force for max pedal deflection : Gain  Gain=force_max_pedal
  Ideal Rotational Motion Sensor : fl_lib/Mechanical/Mechanical Sensors/Ideal Rotational Motion Sensor  offset=0 rad
  Ideal Torque Source : fl_lib/Mechanical/Mechanical Sources/Ideal Torque Source
  Mechanical Rotational Reference : fl_lib/Mechanical/Rotational Elements/Mechanical Rotational Reference
  PS Product : fl_lib/Physical Signals/Functions/PS Product
  Simulink-PS Converter1 : nesl_utility/Simulink-PS Converter  PhysicalDomain=network_engine_domain  SubClassName=ps_input  LeftPortType=input  RightPortType=output  PseudoPeriodic=off  Frequencies=[]  NoiseDistribution=none  NoiseParameters=[]  Unit=N*m  AffineConversion=off  InputFiltering=off  SimscapeFilterOrder=1  InputFilterTimeConstant=0.001  UdotUserProvided=1
  Torque per unit brake pedal force : Gain  Gain=braking_torque_to_pedal_force_ratio
  y=tanh(x) : Subsystem
  R : PMIOPort  Port=1  Side=Right
  wires:
  Pedal/1 -> Force for max pedal deflection/1
  Force for max pedal deflection/1 -> Torque per unit brake pedal force/1
  Torque per unit brake pedal force/1 -> Dead Zone/1
  Dead Zone/1 -> Simulink-PS Converter1/1
  connections:
  y=tanh(x)/RConn1 -- PS Product/LConn2
  Ideal Rotational Motion Sensor/RConn1 -- Mechanical Rotational Reference/LConn1 -- Ideal Torque Source/RConn2
  Ideal Rotational Motion Sensor/LConn1 -- Ideal Torque Source/LConn1 -- R/RConn1
  PS Product/RConn1 -- Ideal Torque Source/RConn1
  Simulink-PS Converter1/RConn1 -- PS Product/LConn1
  Ideal Rotational Motion Sensor/RConn2 -- y=tanh(x)/LConn1

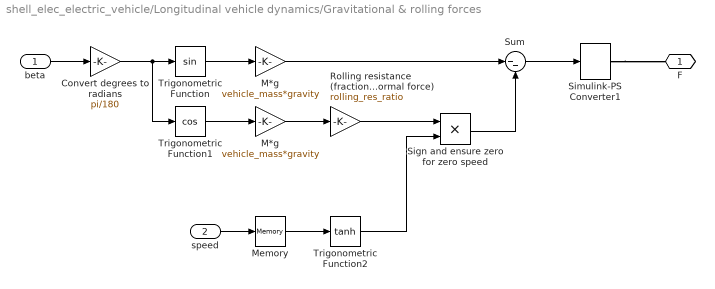
== system shell_elec_electric_vehicle/Longitudinal vehicle dynamics/Gravitational & rolling forces ==
  beta : Inport
  speed : Inport  Port=2
  " M*g " : Gain  Gain=vehicle_mass*gravity
  Convert degrees to radians : Gain  Gain=pi/180
  M*g : Gain  Gain=vehicle_mass*gravity
  Memory : Memory
  Rolling resistance (fraction of normal force) : Gain  Gain=rolling_res_ratio
  Sign and ensure zero for zero speed : Product
  Simulink-PS Converter1 : nesl_utility/Simulink-PS Converter  PhysicalDomain=network_engine_domain  SubClassName=ps_input  LeftPortType=input  RightPortType=output  PseudoPeriodic=off  Frequencies=[]  NoiseDistribution=none  NoiseParameters=[]  Unit=N*m  AffineConversion=off  InputFiltering=off  SimscapeFilterOrder=1  InputFilterTimeConstant=0.001  UdotUserProvided=1
  Sum : Sum  Inputs=|--
  Trigonometric Function : Trigonometry
  Trigonometric Function1 : Trigonometry  Operator=cos
  Trigonometric Function2 : Trigonometry  Operator=tanh
  F : PMIOPort  Port=1  Side=Right
  wires:
  beta/1 -> Convert degrees to radians/1
  Convert degrees to radians/1 -> Trigonometric Function1/1, Trigonometric Function/1
  Trigonometric Function/1 -> " M*g "/1
  Trigonometric Function1/1 -> M*g/1
  M*g/1 -> Rolling resistance (fraction of normal force)/1
  " M*g "/1 -> Sum/1
  Sum/1 -> Simulink-PS Converter1/1
  speed/1 -> Memory/1
  Rolling resistance (fraction of normal force)/1 -> Sign and ensure zero for zero speed/1
  Trigonometric Function2/1 -> Sign and ensure zero for zero speed/2
  Memory/1 -> Trigonometric Function2/1
  Sign and ensure zero for zero speed/1 -> Sum/2
  connections:
  Simulink-PS Converter1/RConn1 -- F/RConn1

== system shell_elec_electric_vehicle/Longitudinal vehicle dynamics/Measurement ==
  Ideal Translational Motion Sensor : fl_lib/Mechanical/Mechanical Sensors/Ideal Translational Motion Sensor  offset=0 m
  Mechanical Translational Reference : fl_lib/Mechanical/Translational Elements/Mechanical Translational Reference
  PS-Simulink Converter3 : nesl_utility/PS-Simulink Converter  PhysicalDomain=network_engine_domain  SubClassName=ps_output  LeftPortType=input  RightPortType=output  PseudoPeriodic=off  Frequencies=[]  Unit=mph  AffineConversion=off
  R : PMIOPort  Port=1  Side=Left
  w : PMIOPort  Port=2  Side=Right
  speed : Outport
  tag scope: vehicleVelocity=global
  wires:
  PS-Simulink Converter3/1 -> speed/1, [vehicleVelocity]  "MPH"
  connections:
  R/RConn1 -- Ideal Translational Motion Sensor/LConn1
  Mechanical Translational Reference/LConn1 -- Ideal Translational Motion Sensor/RConn1
  Ideal Translational Motion Sensor/RConn2 -- PS-Simulink Converter3/LConn1 -- w/RConn1

== system shell_elec_electric_vehicle/Vehicle control system/Add feedforward term to counter effect of gravity when on an incline. Results in regenerative braking when moving downhill. ==
  inclinometer : Inport
  " M " : Gain  Gain=vehicle_mass
  1/ratio : Gain  Gain=1/gear_ratio
  Wheel radius : Gain  Gain=wheel_radius
  feedforward torque : Outport
  wires:
  inclinometer/1 -> " M "/1
  " M "/1 -> Wheel radius/1
  Wheel radius/1 -> 1/ratio/1  "Wheel torque"
  1/ratio/1 -> feedforward torque/1  "Motor torque"

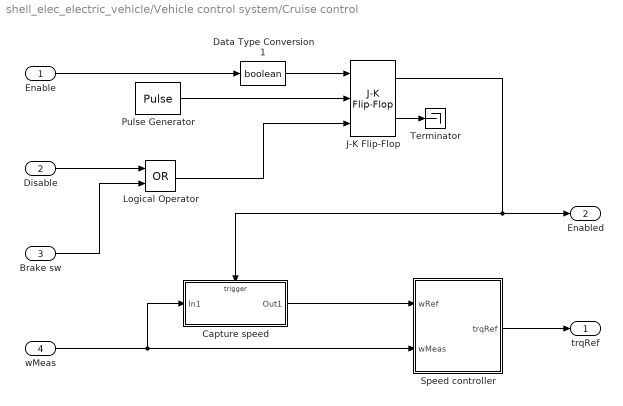
== system shell_elec_electric_vehicle/Vehicle control system/Cruise control ==
  Enable : Inport
  Disable : Inport  Port=2
  Brake sw : Inport  Port=3
  wMeas : Inport  Port=4
  Capture speed : Subsystem  TreatAsAtomicUnit=on
  Data Type Conversion1 : DataTypeConversion  OutDataTypeStr=boolean
  J-K Flip-Flop : simulink_extras/Flip Flops/J-K Flip-Flop  initial_condition=0
  Logical Operator : Logic  Operator=OR  AllPortsSameDT=off  OutDataTypeStr=boolean
  Pulse Generator : DiscretePulseGenerator  Period=10  PulseWidth=5  SampleTime=0.01
  Speed controller : Subsystem  mask(P+I motor speed controller){Kp=100, Ki=100, trqMax=max_torque, ts=dt}
      mask prompts: Kp "Proportional gain (Nm/(rad/s))"; Ki "Integral gain (Nm/rad)"; trqMax "Maximum torque demand"; ts "Sample time"
      mask help: Inputs wRef and wMeas are the demanded rotor speed and measured rotor speed in rad/s. The controller output is a torque demand in Nm.
  Terminator : Terminator
  trqRef : Outport
  Enabled : Outport  Port=2
  wires:
  Enable/1 -> Data Type Conversion1/1
  Pulse Generator/1 -> J-K Flip-Flop/2
  Disable/1 -> Logical Operator/1
  Speed controller/1(trqRef) -> trqRef/1
  Brake sw/1 -> Logical Operator/2
  wMeas/1 -> Capture speed/1(In1), Speed controller/2(wMeas)
  Logical Operator/1 -> J-K Flip-Flop/3
  J-K Flip-Flop/1 -> Capture speed/Trigger, Enabled/1
  Data Type Conversion1/1 -> J-K Flip-Flop/1
  J-K Flip-Flop/2 -> Terminator/1
  Capture speed/1(Out1) -> Speed controller/1(wRef)

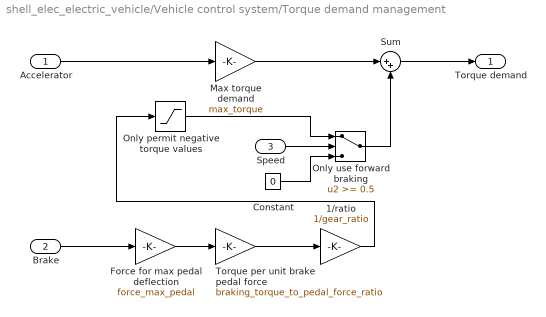
== system shell_elec_electric_vehicle/Vehicle control system/Torque demand management ==
  Accelerator : Inport
  Brake : Inport  Port=2
  Speed : Inport  Port=3
  1/ratio : Gain  Gain=1/gear_ratio
  Constant : Constant  Value=0  SampleTime=dt
  Force for max pedal deflection : Gain  Gain=force_max_pedal
  Max torque demand : Gain  Gain=max_torque
  Only permit negative torque values : Saturate  UpperLimit=-10  LowerLimit=-max_torque
  Only use forward braking : Switch  Threshold=0.5  InputSameDT=on
  Sum : Sum  Inputs=|++
  Torque per unit brake pedal force : Gain  Gain=braking_torque_to_pedal_force_ratio
  Torque demand : Outport
  wires:
  Max torque demand/1 -> Sum/1
  Brake/1 -> Force for max pedal deflection/1
  Sum/1 -> Torque demand/1
  Accelerator/1 -> Max torque demand/1
  Torque per unit brake pedal force/1 -> 1/ratio/1
  1/ratio/1 -> Only permit negative torque values/1
  Force for max pedal deflection/1 -> Torque per unit brake pedal force/1
  Speed/1 -> Only use forward braking/2
  Only use forward braking/1 -> Sum/2
  Constant/1 -> Only use forward braking/3
  Only permit negative torque values/1 -> Only use forward braking/1

== system shell_elec_electric_vehicle/Longitudinal vehicle dynamics/Aerodynamic drag/y=tanh(x) ==
  1 : fl_lib/Physical Signals/Sources/PS Constant  constant=1
  2 : fl_lib/Physical Signals/Functions/PS Gain  gain=2
  exp(2x) : fl_lib/Physical Signals/Functions/PS Math Function  fcn_choice=3
  exp(2x)+1 : fl_lib/Physical Signals/Functions/PS Add
  exp(2x)-1 : fl_lib/Physical Signals/Functions/PS Subtract
  tanh(x) : fl_lib/Physical Signals/Functions/PS Divide
  x : PMIOPort  Port=1  Side=Left
  y : PMIOPort  Port=2  Side=Right
  connections:
  y/RConn1 -- tanh(x)/RConn1
  x/RConn1 -- 2/LConn1
  exp(2x)-1/RConn1 -- tanh(x)/LConn1
  exp(2x)+1/RConn1 -- tanh(x)/LConn2
  exp(2x)+1/LConn2 -- exp(2x)-1/LConn1 -- exp(2x)/RConn1
  2/RConn1 -- exp(2x)/LConn1
  exp(2x)-1/LConn2 -- exp(2x)+1/LConn1 -- 1/RConn1

== system shell_elec_electric_vehicle/Longitudinal vehicle dynamics/Braking torque/y=tanh(x) ==
  1 : fl_lib/Physical Signals/Sources/PS Constant  constant=1
  2 : fl_lib/Physical Signals/Functions/PS Gain  gain=2
  exp(2x) : fl_lib/Physical Signals/Functions/PS Math Function  fcn_choice=3
  exp(2x)+1 : fl_lib/Physical Signals/Functions/PS Add
  exp(2x)-1 : fl_lib/Physical Signals/Functions/PS Subtract
  tanh(x) : fl_lib/Physical Signals/Functions/PS Divide
  x : PMIOPort  Port=1  Side=Left
  y : PMIOPort  Port=2  Side=Right
  connections:
  y/RConn1 -- tanh(x)/RConn1
  x/RConn1 -- 2/LConn1
  exp(2x)-1/RConn1 -- tanh(x)/LConn1
  exp(2x)+1/RConn1 -- tanh(x)/LConn2
  exp(2x)+1/LConn2 -- exp(2x)-1/LConn1 -- exp(2x)/RConn1
  2/RConn1 -- exp(2x)/LConn1
  exp(2x)-1/LConn2 -- exp(2x)+1/LConn1 -- 1/RConn1

== system shell_elec_electric_vehicle/Vehicle control system/Cruise control/Capture speed ==
  In1 : Inport
  Trigger : TriggerPort  VariantControl=Variant
  Out1 : Outport
  wires:
  In1/1 -> Out1/1

== system shell_elec_electric_vehicle/Vehicle control system/Cruise control/Speed controller ==
  wRef : Inport
  wMeas : Inport  Port=2
  Add : Sum  Inputs=|+-
  Add1 : Sum
  Discrete-Time Integrator : DiscreteIntegrator  gainval=Ki  SampleTime=ts  LimitOutput=on  UpperSaturationLimit=trqMax  LowerSaturationLimit=-trqMax  ICPrevOutput=DiscIntNeverNeededParam  ICPrevScaledInput=DiscIntNeverNeededParam
  Kp : Gain  Gain=Kp
  trqRef : Outport
  wires:
  wRef/1 -> Add/1
  Kp/1 -> Add1/1
  Discrete-Time Integrator/1 -> Add1/2
  wMeas/1 -> Add/2
  Add1/1 -> trqRef/1
  Add/1 -> Kp/1, Discrete-Time Integrator/1
